simulink model "Last_version_po_STO"  (R2018a)
settings: Solver=FixedStepAuto  StartTime=0.0  StopTime=inf  FixedStep=1e-3  MaxStep=1e-4  RelTol=1e-3
undefined symbols (not defined in the file): D11, Delta
libraries: powerlib x118, simulink_extras x25, powerlib_meascontrol x18, simulink x8, xpcutilitieslib x2, xpcrtudplib x2, opclib x1, sldrtlib x1
(part 3 of 3)

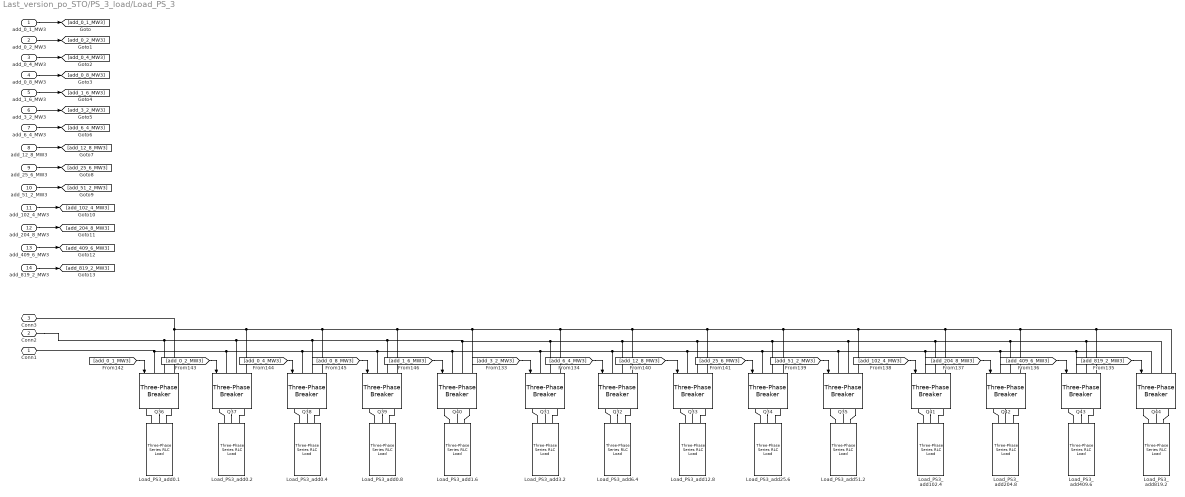
== system Last_version_po_STO/PS_3_load/Load_PS_3 ==
  add_0_1_MW3 : Inport
  add_0_2_MW3 : Inport  Port=2
  add_0_4_MW3 : Inport  Port=3
  add_0_8_MW3 : Inport  Port=4
  add_1_6_MW3 : Inport  Port=5
  add_3_2_MW3 : Inport  Port=6
  add_6_4_MW3 : Inport  Port=7
  add_12_8_MW3 : Inport  Port=8
  add_25_6_MW3 : Inport  Port=9
  add_51_2_MW3 : Inport  Port=10
  add_102_4_MW3 : Inport  Port=11
  add_204_8_MW3 : Inport  Port=12
  add_409_6_MW3 : Inport  Port=13
  add_819_2_MW3 : Inport  Port=14
  Load_PS3_add0.1 : powerlib/Elements/Three-Phase Series RLC Load  LConnTagsString=A|B|C  Configuration=Y (grounded)  NominalVoltage=110e3  Vabc=[1e3 1e3 1e3]  Vabcp=[1e3 1e3 1e3]  NominalFrequency=50  UnbalancedPower=off  ActivePower=0.1e6  InductivePower=0  CapacitivePower=0  Pabc=[10e3 9e3 11e3]  QLabc=[100 90 110]  QCabc=[100 90 110]  Pabcp=[10e3 9e3 11e3]  QLabcp=[100 90 110]  QCabcp=[100 90 110]  Measurements=None  LoadType=constant Z
      settings: SourceProductName=Simscape Electrical
  Load_PS3_add0.2 : powerlib/Elements/Three-Phase Series RLC Load  LConnTagsString=A|B|C  Configuration=Y (grounded)  NominalVoltage=110e3  Vabc=[1e3 1e3 1e3]  Vabcp=[1e3 1e3 1e3]  NominalFrequency=50  UnbalancedPower=off  ActivePower=0.2e6  InductivePower=0  CapacitivePower=0  Pabc=[10e3 9e3 11e3]  QLabc=[100 90 110]  QCabc=[100 90 110]  Pabcp=[10e3 9e3 11e3]  QLabcp=[100 90 110]  QCabcp=[100 90 110]  Measurements=None  LoadType=constant Z
      settings: SourceProductName=Simscape Electrical
  Load_PS3_add0.4 : powerlib/Elements/Three-Phase Series RLC Load  LConnTagsString=A|B|C  Configuration=Y (grounded)  NominalVoltage=110e3  Vabc=[1e3 1e3 1e3]  Vabcp=[1e3 1e3 1e3]  NominalFrequency=50  UnbalancedPower=off  ActivePower=0.4e6  InductivePower=0  CapacitivePower=0  Pabc=[10e3 9e3 11e3]  QLabc=[100 90 110]  QCabc=[100 90 110]  Pabcp=[10e3 9e3 11e3]  QLabcp=[100 90 110]  QCabcp=[100 90 110]  Measurements=None  LoadType=constant Z
      settings: SourceProductName=Simscape Electrical
  Load_PS3_add0.8 : powerlib/Elements/Three-Phase Series RLC Load  LConnTagsString=A|B|C  Configuration=Y (grounded)  NominalVoltage=110e3  Vabc=[1e3 1e3 1e3]  Vabcp=[1e3 1e3 1e3]  NominalFrequency=50  UnbalancedPower=off  ActivePower=0.8e6  InductivePower=0  CapacitivePower=0  Pabc=[10e3 9e3 11e3]  QLabc=[100 90 110]  QCabc=[100 90 110]  Pabcp=[10e3 9e3 11e3]  QLabcp=[100 90 110]  QCabcp=[100 90 110]  Measurements=None  LoadType=constant Z
      settings: SourceProductName=Simscape Electrical
  Load_PS3_add1.6 : powerlib/Elements/Three-Phase Series RLC Load  LConnTagsString=A|B|C  Configuration=Y (grounded)  NominalVoltage=110e3  Vabc=[1e3 1e3 1e3]  Vabcp=[1e3 1e3 1e3]  NominalFrequency=50  UnbalancedPower=off  ActivePower=1.6e6  InductivePower=0  CapacitivePower=0  Pabc=[10e3 9e3 11e3]  QLabc=[100 90 110]  QCabc=[100 90 110]  Pabcp=[10e3 9e3 11e3]  QLabcp=[100 90 110]  QCabcp=[100 90 110]  Measurements=None  LoadType=constant Z
      settings: SourceProductName=Simscape Electrical
  Load_PS3_add102.4 : powerlib/Elements/Three-Phase Series RLC Load  LConnTagsString=A|B|C  Configuration=Y (grounded)  NominalVoltage=110e3  Vabc=[1e3 1e3 1e3]  Vabcp=[1e3 1e3 1e3]  NominalFrequency=50  UnbalancedPower=off  ActivePower=102.4e6  InductivePower=0  CapacitivePower=0  Pabc=[10e3 9e3 11e3]  QLabc=[100 90 110]  QCabc=[100 90 110]  Pabcp=[10e3 9e3 11e3]  QLabcp=[100 90 110]  QCabcp=[100 90 110]  Measurements=None  LoadType=constant Z
      settings: SourceProductName=Simscape Electrical
  Load_PS3_add12.8 : powerlib/Elements/Three-Phase Series RLC Load  LConnTagsString=A|B|C  Configuration=Y (grounded)  NominalVoltage=110e3  Vabc=[1e3 1e3 1e3]  Vabcp=[1e3 1e3 1e3]  NominalFrequency=50  UnbalancedPower=off  ActivePower=12.8e6  InductivePower=0  CapacitivePower=0  Pabc=[10e3 9e3 11e3]  QLabc=[100 90 110]  QCabc=[100 90 110]  Pabcp=[10e3 9e3 11e3]  QLabcp=[100 90 110]  QCabcp=[100 90 110]  Measurements=None  LoadType=constant Z
      settings: SourceProductName=Simscape Electrical
  Load_PS3_add204.8 : powerlib/Elements/Three-Phase Series RLC Load  LConnTagsString=A|B|C  Configuration=Y (grounded)  NominalVoltage=110e3  Vabc=[1e3 1e3 1e3]  Vabcp=[1e3 1e3 1e3]  NominalFrequency=50  UnbalancedPower=off  ActivePower=204.8e6  InductivePower=0  CapacitivePower=0  Pabc=[10e3 9e3 11e3]  QLabc=[100 90 110]  QCabc=[100 90 110]  Pabcp=[10e3 9e3 11e3]  QLabcp=[100 90 110]  QCabcp=[100 90 110]  Measurements=None  LoadType=constant Z
      settings: SourceProductName=Simscape Electrical
  Load_PS3_add25.6 : powerlib/Elements/Three-Phase Series RLC Load  LConnTagsString=A|B|C  Configuration=Y (grounded)  NominalVoltage=110e3  Vabc=[1e3 1e3 1e3]  Vabcp=[1e3 1e3 1e3]  NominalFrequency=50  UnbalancedPower=off  ActivePower=25.6e6  InductivePower=0  CapacitivePower=0  Pabc=[10e3 9e3 11e3]  QLabc=[100 90 110]  QCabc=[100 90 110]  Pabcp=[10e3 9e3 11e3]  QLabcp=[100 90 110]  QCabcp=[100 90 110]  Measurements=None  LoadType=constant Z
      settings: SourceProductName=Simscape Electrical
  Load_PS3_add3.2 : powerlib/Elements/Three-Phase Series RLC Load  LConnTagsString=A|B|C  Configuration=Y (grounded)  NominalVoltage=110e3  Vabc=[1e3 1e3 1e3]  Vabcp=[1e3 1e3 1e3]  NominalFrequency=50  UnbalancedPower=off  ActivePower=3.2e6  InductivePower=0  CapacitivePower=0  Pabc=[10e3 9e3 11e3]  QLabc=[100 90 110]  QCabc=[100 90 110]  Pabcp=[10e3 9e3 11e3]  QLabcp=[100 90 110]  QCabcp=[100 90 110]  Measurements=None  LoadType=constant Z
      settings: SourceProductName=Simscape Electrical
  Load_PS3_add409.6 : powerlib/Elements/Three-Phase Series RLC Load  LConnTagsString=A|B|C  Configuration=Y (grounded)  NominalVoltage=110e3  Vabc=[1e3 1e3 1e3]  Vabcp=[1e3 1e3 1e3]  NominalFrequency=50  UnbalancedPower=off  ActivePower=409.6e6  InductivePower=0  CapacitivePower=0  Pabc=[10e3 9e3 11e3]  QLabc=[100 90 110]  QCabc=[100 90 110]  Pabcp=[10e3 9e3 11e3]  QLabcp=[100 90 110]  QCabcp=[100 90 110]  Measurements=None  LoadType=constant Z
      settings: SourceProductName=Simscape Electrical
  Load_PS3_add51.2 : powerlib/Elements/Three-Phase Series RLC Load  LConnTagsString=A|B|C  Configuration=Y (grounded)  NominalVoltage=110e3  Vabc=[1e3 1e3 1e3]  Vabcp=[1e3 1e3 1e3]  NominalFrequency=50  UnbalancedPower=off  ActivePower=51.2e6  InductivePower=0  CapacitivePower=0  Pabc=[10e3 9e3 11e3]  QLabc=[100 90 110]  QCabc=[100 90 110]  Pabcp=[10e3 9e3 11e3]  QLabcp=[100 90 110]  QCabcp=[100 90 110]  Measurements=None  LoadType=constant Z
      settings: SourceProductName=Simscape Electrical
  Load_PS3_add6.4 : powerlib/Elements/Three-Phase Series RLC Load  LConnTagsString=A|B|C  Configuration=Y (grounded)  NominalVoltage=110e3  Vabc=[1e3 1e3 1e3]  Vabcp=[1e3 1e3 1e3]  NominalFrequency=50  UnbalancedPower=off  ActivePower=6.4e6  InductivePower=0  CapacitivePower=0  Pabc=[10e3 9e3 11e3]  QLabc=[100 90 110]  QCabc=[100 90 110]  Pabcp=[10e3 9e3 11e3]  QLabcp=[100 90 110]  QCabcp=[100 90 110]  Measurements=None  LoadType=constant Z
      settings: SourceProductName=Simscape Electrical
  Load_PS3_add819.2 : powerlib/Elements/Three-Phase Series RLC Load  LConnTagsString=A|B|C  Configuration=Y (grounded)  NominalVoltage=110e3  Vabc=[1e3 1e3 1e3]  Vabcp=[1e3 1e3 1e3]  NominalFrequency=50  UnbalancedPower=off  ActivePower=819.2e6  InductivePower=0  CapacitivePower=0  Pabc=[10e3 9e3 11e3]  QLabc=[100 90 110]  QCabc=[100 90 110]  Pabcp=[10e3 9e3 11e3]  QLabcp=[100 90 110]  QCabcp=[100 90 110]  Measurements=None  LoadType=constant Z
      settings: SourceProductName=Simscape Electrical
  Q{31..44} (14 alike) : powerlib/Elements/Three-Phase Breaker  InitialState=open  SwitchA=on  SwitchB=on  SwitchC=on  SwitchTimes="[1/60  5/60]"  External=on  BreakerResistance=0.01  SnubberResistance=1e6  SnubberCapacitance=inf  Measurements=None
      settings: SourceProductName=Simscape Electrical
  Conn1 : PMIOPort  Side=Left
  Conn2 : PMIOPort  Port=2  Side=Left
  Conn3 : PMIOPort  Port=3  Side=Left
  wires:
  [add_0_2_MW3] -> Q37/1
  [add_12_8_MW3] -> Q33/1
  [add_0_4_MW3] -> Q38/1
  [add_102_4_MW3] -> Q41/1
  [add_25_6_MW3] -> Q34/1
  [add_409_6_MW3] -> Q43/1
  [add_819_2_MW3] -> Q44/1
  [add_6_4_MW3] -> Q32/1
  [add_3_2_MW3] -> Q31/1
  [add_0_8_MW3] -> Q39/1
  [add_1_6_MW3] -> Q40/1
  [add_0_1_MW3] -> Q36/1
  [add_204_8_MW3] -> Q42/1
  [add_51_2_MW3] -> Q35/1
  add_0_1_MW3/1 -> [add_0_1_MW3]
  add_0_2_MW3/1 -> [add_0_2_MW3]
  add_0_4_MW3/1 -> [add_0_4_MW3]
  add_0_8_MW3/1 -> [add_0_8_MW3]
  add_1_6_MW3/1 -> [add_1_6_MW3]
  add_3_2_MW3/1 -> [add_3_2_MW3]
  add_6_4_MW3/1 -> [add_6_4_MW3]
  add_12_8_MW3/1 -> [add_12_8_MW3]
  add_25_6_MW3/1 -> [add_25_6_MW3]
  add_51_2_MW3/1 -> [add_51_2_MW3]
  add_102_4_MW3/1 -> [add_102_4_MW3]
  add_204_8_MW3/1 -> [add_204_8_MW3]
  add_409_6_MW3/1 -> [add_409_6_MW3]
  add_819_2_MW3/1 -> [add_819_2_MW3]
  connections:
  Load_PS3_add0.8/LConn1 -- Q39/RConn1
  Load_PS3_add12.8/LConn3 -- Q33/RConn3
  Q43/LConn3 -- Q44/LConn3 -- Q42/LConn3 -- Q41/LConn3 -- Q35/LConn3 -- Q34/LConn3 -- Q33/LConn3 -- Q32/LConn3 -- Q31/LConn3 -- Q40/LConn3 -- Conn3/RConn1 -- Q36/LConn3 -- Q37/LConn3 -- Q38/LConn3 -- Q39/LConn3
  Q43/LConn2 -- Q44/LConn2 -- Q42/LConn2 -- Q41/LConn2 -- Q35/LConn2 -- Q34/LConn2 -- Q33/LConn2 -- Q32/LConn2 -- Q31/LConn2 -- Q40/LConn2 -- Conn2/RConn1 -- Q36/LConn2 -- Q37/LConn2 -- Q38/LConn2 -- Q39/LConn2
  Q43/LConn1 -- Q44/LConn1 -- Q42/LConn1 -- Q41/LConn1 -- Q35/LConn1 -- Q34/LConn1 -- Q33/LConn1 -- Q32/LConn1 -- Q31/LConn1 -- Q40/LConn1 -- Conn1/RConn1 -- Q36/LConn1 -- Q37/LConn1 -- Q38/LConn1 -- Q39/LConn1
  Q41/RConn2 -- Load_PS3_add102.4/LConn2
  Load_PS3_add12.8/LConn2 -- Q33/RConn2
  Load_PS3_add409.6/LConn1 -- Q43/RConn1
  Q44/RConn1 -- Load_PS3_add819.2/LConn1
  Load_PS3_add12.8/LConn1 -- Q33/RConn1
  Load_PS3_add6.4/LConn3 -- Q32/RConn3
  Load_PS3_add51.2/LConn2 -- Q35/RConn2
  Q34/RConn2 -- Load_PS3_add25.6/LConn2
  Q35/RConn1 -- Load_PS3_add51.2/LConn1
  Load_PS3_add1.6/LConn2 -- Q40/RConn2
  Load_PS3_add25.6/LConn3 -- Q34/RConn3
  Q35/RConn3 -- Load_PS3_add51.2/LConn3
  Load_PS3_add0.8/LConn3 -- Q39/RConn3
  Load_PS3_add102.4/LConn3 -- Q41/RConn3
  Load_PS3_add0.4/LConn3 -- Q38/RConn3
  Load_PS3_add0.4/LConn2 -- Q38/RConn2
  Load_PS3_add0.4/LConn1 -- Q38/RConn1
  Q37/RConn2 -- Load_PS3_add0.2/LConn2
  Q36/RConn2 -- Load_PS3_add0.1/LConn2
  Load_PS3_add0.2/LConn3 -- Q37/RConn3
  Q32/RConn2 -- Load_PS3_add6.4/LConn2
  Q44/RConn3 -- Load_PS3_add819.2/LConn3
  Load_PS3_add6.4/LConn1 -- Q32/RConn1
  Load_PS3_add819.2/LConn2 -- Q44/RConn2
  Q39/RConn2 -- Load_PS3_add0.8/LConn2
  Load_PS3_add204.8/LConn3 -- Q42/RConn3
  Load_PS3_add3.2/LConn3 -- Q31/RConn3
  Load_PS3_add0.1/LConn3 -- Q36/RConn3
  Load_PS3_add25.6/LConn1 -- Q34/RConn1
  Load_PS3_add3.2/LConn2 -- Q31/RConn2
  Load_PS3_add3.2/LConn1 -- Q31/RConn1
  Load_PS3_add102.4/LConn1 -- Q41/RConn1
  Q40/RConn1 -- Load_PS3_add1.6/LConn1
  Q40/RConn3 -- Load_PS3_add1.6/LConn3
  Load_PS3_add0.1/LConn1 -- Q36/RConn1
  Q43/RConn2 -- Load_PS3_add409.6/LConn2
  Load_PS3_add409.6/LConn3 -- Q43/RConn3
  Load_PS3_add204.8/LConn1 -- Q42/RConn1
  Load_PS3_add204.8/LConn2 -- Q42/RConn2
  Load_PS3_add0.2/LConn1 -- Q37/RConn1

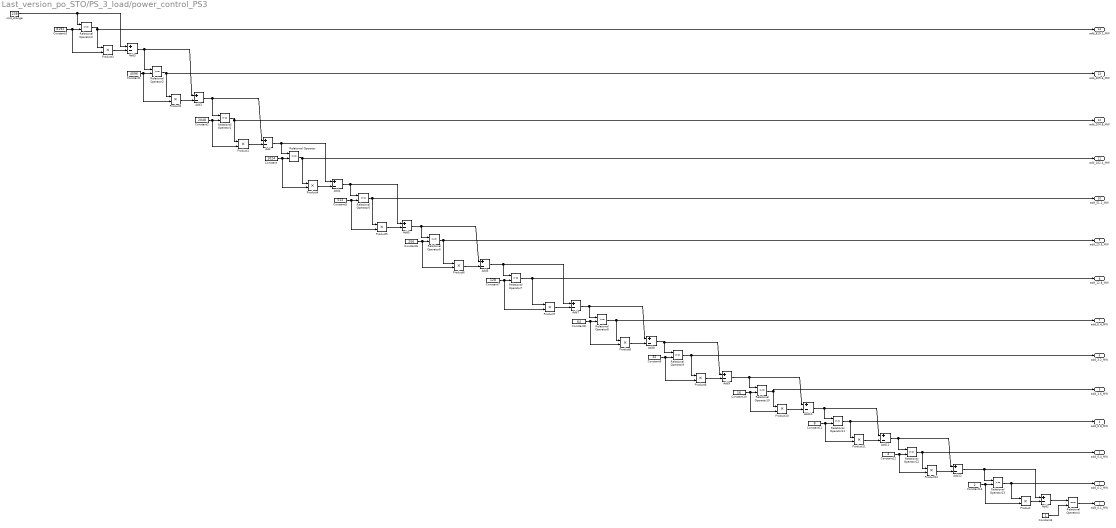
== system Last_version_po_STO/PS_3_load/power_control_PS3 ==
  Add{,1..12} (13 alike) : Sum  Inputs=+-
  Constant : Constant  Value=1024
  Constant1 : Constant  Value=4096
  Constant10 : Constant  Value=16
  Constant11 : Constant  Value=8
  Constant12 : Constant  Value=4
  Constant13 : Constant  Value=2
  Constant2 : Constant  Value=2048
  Constant3 : Constant  Value=8192
  Constant4 : Constant
  Constant5 : Constant  Value=512
  Constant6 : Constant  Value=256
  Constant7 : Constant  Value=128
  Constant8 : Constant  Value=64
  Constant9 : Constant  Value=32
  Product{,1..12} (13 alike) : Product
  Relational Operator{,1..3,5..13} (13 alike) : RelationalOperator  OutDataTypeStr=boolean  RndMeth=Simplest
  Relational Operator4 : RelationalOperator  Operator===  OutDataTypeStr=boolean  RndMeth=Simplest
  cnst_change : Constant  Value=238
  add_0.1_MW : Outport
  add_0.2_MW : Outport  Port=2
  add_0.4_MW : Outport  Port=3
  add_0.8_MW : Outport  Port=4
  add_1.6_MW : Outport  Port=5
  add_3.2_MW : Outport  Port=6
  add_6.4_MW : Outport  Port=7
  add_12.8_MW : Outport  Port=8
  add_25.6_MW : Outport  Port=9
  add_51.2_MW : Outport  Port=10
  add_102.4_MW : Outport  Port=11
  add_204.8_MW : Outport  Port=12
  add_409.6_MW : Outport  Port=13
  add_819.2_MW : Outport  Port=14
  wires:
  Relational Operator13/1 -> Product/1, add_0.2_MW/1
  Relational Operator12/1 -> Product12/1, add_0.4_MW/1
  Relational Operator11/1 -> Product11/1, add_0.8_MW/1
  Relational Operator10/1 -> Product10/1, add_1.6_MW/1
  Relational Operator9/1 -> Product9/1, add_3.2_MW/1
  Relational Operator8/1 -> Product8/1, add_6.4_MW/1
  Relational Operator7/1 -> Product7/1, add_12.8_MW/1
  Product12/1 -> Add12/2
  Add12/1 -> Relational Operator13/1, Add2/1
  Constant13/1 -> Relational Operator13/2, Product/2
  Constant12/1 -> Relational Operator12/2, Product12/2
  Add11/1 -> Relational Operator12/1, Add12/1
  Product11/1 -> Add11/2
  Product10/1 -> Add10/2
  Add10/1 -> Relational Operator11/1, Add11/1
  Constant11/1 -> Relational Operator11/2, Product11/2
  Constant10/1 -> Relational Operator10/2, Product10/2
  Add9/1 -> Relational Operator10/1, Add10/1
  Product9/1 -> Add9/2
  Product8/1 -> Add8/2
  Add8/1 -> Relational Operator9/1, Add9/1
  Constant9/1 -> Relational Operator9/2, Product9/2
  Constant8/1 -> Relational Operator8/2, Product8/2
  Add7/1 -> Relational Operator8/1, Add8/1
  Product7/1 -> Add7/2
  Relational Operator6/1 -> Product6/1, add_25.6_MW/1
  Relational Operator5/1 -> add_51.2_MW/1, Product5/1
  Product6/1 -> Add6/2
  Add6/1 -> Relational Operator7/1, Add7/1
  Constant7/1 -> Relational Operator7/2, Product7/2
  Constant6/1 -> Relational Operator6/2, Product6/2
  Add5/1 -> Add6/1, Relational Operator6/1
  Product5/1 -> Add5/2
  Product4/1 -> Add4/2
  Add4/1 -> Relational Operator5/1, Add5/1
  Constant5/1 -> Relational Operator5/2, Product5/2
  Relational Operator3/1 -> add_819.2_MW/1, Product3/1
  Add3/1 -> Add1/1, Relational Operator2/1
  Product3/1 -> Add3/2
  Constant/1 -> Relational Operator/2, Product4/2
  Relational Operator1/1 -> add_204.8_MW/1, Product1/1
  Constant2/1 -> Product1/2, Relational Operator1/2
  Relational Operator/1 -> Product4/1, add_102.4_MW/1
  Add/1 -> Relational Operator/1, Add4/1
  Product/1 -> Add2/2
  Product1/1 -> Add/2
  Constant4/1 -> Relational Operator4/2
  Relational Operator4/1 -> add_0.1_MW/1
  cnst_change/1 -> Add3/1, Relational Operator3/1
  Product2/1 -> Add1/2
  Constant1/1 -> Product2/2, Relational Operator2/2
  Add1/1 -> Add/1, Relational Operator1/1
  Relational Operator2/1 -> add_409.6_MW/1, Product2/1
  Add2/1 -> Relational Operator4/1
  Constant3/1 -> Product3/2, Relational Operator3/2

== system Last_version_po_STO/choosing_PO/pulse_limited ==
  In : Inport
  t_pulse : Inport  Port=2
  Delay1 : Delay  DelayLength=1  InitialCondition=0
  Detect Increase : simulink/Logic and Bit Operations/Detect Increase  vinit=0.0  OutDataTypeStr=boolean
  S-R Flip-Flop : simulink_extras/Flip Flops/S-R Flip-Flop  initial_condition=0
  Terminator : Terminator
  relay_t1 : Subsystem
  Out : Outport
  wires:
  relay_t1/1(Out) -> Delay1/1
  S-R Flip-Flop/1 -> Out/1, relay_t1/1(In)
  Delay1/1 -> S-R Flip-Flop/2
  Detect Increase/1 -> S-R Flip-Flop/1
  [t_pulse] -> relay_t1/2(t_vv)
  In/1 -> Detect Increase/1
  S-R Flip-Flop/2 -> Terminator/1
  t_pulse/1 -> [t_pulse]

== system Last_version_po_STO/choosing_PO/pulse_limited/relay_t1 ==
  In : Inport
  t_vv : Inport  Port=2
  Data Type Conversion : DataTypeConversion  OutDataTypeStr=double
  Integrator1 : Integrator  ExternalReset=rising  LimitOutput=on  UpperSaturationLimit=10000
  Logical Operator2 : Logic  Operator=NOT  AllPortsSameDT=off  OutDataTypeStr=boolean
  Relational Operator : RelationalOperator  Operator=>  OutDataTypeStr=boolean  RndMeth=Nearest
  Out : Outport
  wires:
  Data Type Conversion/1 -> Integrator1/1
  t_vv/1 -> Relational Operator/2
  Integrator1/1 -> Relational Operator/1
  Relational Operator/1 -> Out/1
  In/1 -> Logical Operator2/1, Data Type Conversion/1
  Logical Operator2/1 -> Integrator1/2
